simulink subsystem "Vehicle_plant_model"  (R2024b)
settings: Solver=VariableStepAuto  StartTime=0.0  StopTime=10.0  RelTol=1e-3
values from neighbouring files (symbols this model uses):
  div_min_MPC = 0.001    [sim_data_vehicle.sldd]    (also in sim_data_vehicle_nl.sldd)
  TimeStep = 0.01    [sim_data_DCmotor_system.sldd]    (also in sim_data_unstable_system.sldd = 0.01
undefined symbols (not defined in the file or in its folder): DiscIntNeverNeededParam, I_val, K_f_val, K_r_val, l_f_val, l_r_val, m_val, x0
settings Model: Creator=tshintai  LastModifiedBy=tshintai
settings SolverCC: AlgebraicLoopSolver=TrustRegion
settings OptimizationCC: ReuseModelBlockBuffer=off
settings DebuggingCC: UnconnectedInputMsg=warning  UnconnectedOutputMsg=warning  UnconnectedLineMsg=warning
settings ModelReferenceCC: EnableRefExpFcnMdlSchedulingChecks=on
settings RTWCC: GPUComputeCapability=3.5  DLArmComputeVersion=19.05

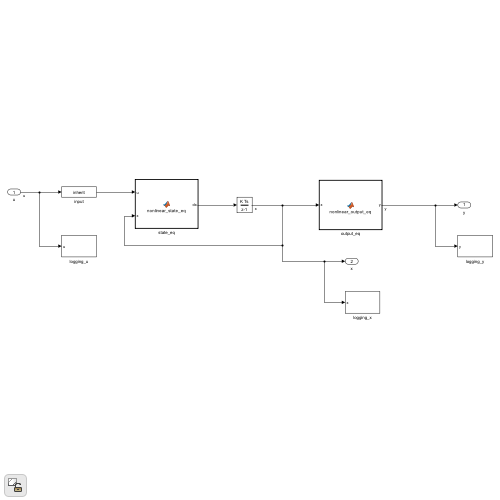
[thumbnail: Simulink's stored preview of the top-level diagram]
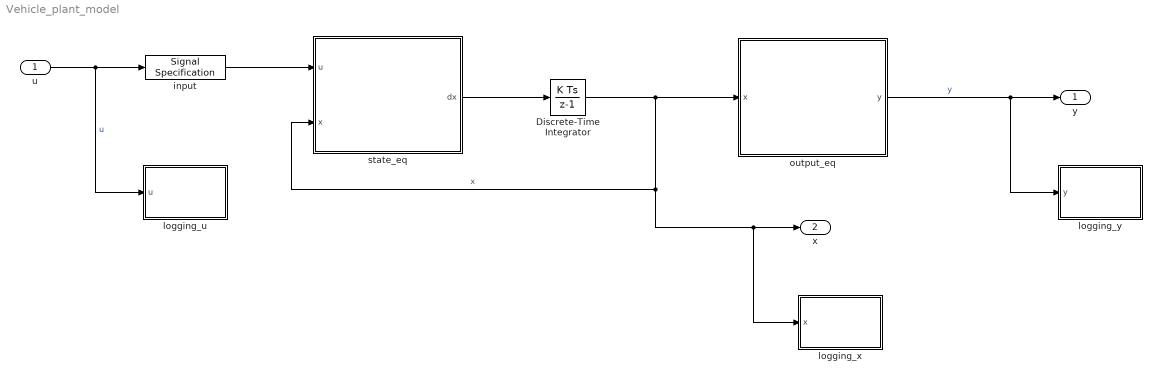
== system Vehicle_plant_model ==
  u : Inport
  Discrete-Time Integrator : DiscreteIntegrator  InitialCondition=x0  SampleTime=TimeStep  ICPrevOutput=DiscIntNeverNeededParam  ICPrevScaledInput=DiscIntNeverNeededParam
  input : SignalSpecification
  logging_u : Subsystem
  logging_x : Subsystem
  logging_y : Subsystem
  output_eq : MATLAB Function  TreatAsAtomicUnit=on
  state_eq : MATLAB Function  TreatAsAtomicUnit=on
  y : Outport
  x : Outport  Port=2
  wires:
  state_eq/1(dx) -> Discrete-Time Integrator/1
  u/1 -> input/1, logging_u/1(u)  "u"
  input/1 -> state_eq/1(u)
  output_eq/1(y) -> logging_y/1(y), y/1  "y"
  Discrete-Time Integrator/1 -> x/1, logging_x/1(x), state_eq/2(x), output_eq/1(x)  "x"

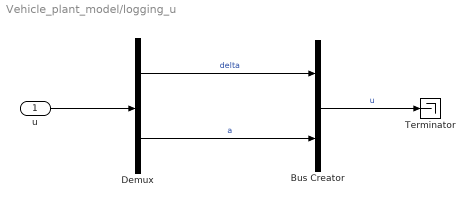
== system Vehicle_plant_model/logging_u ==
  u : Inport
  Bus Creator : BusCreator  Inputs=2
  Demux : Demux  Outputs=2
  Terminator : Terminator
  wires:
  Demux/1 -> Bus Creator/1  "delta"
  u/1 -> Demux/1
  Demux/2 -> Bus Creator/2  "a"
  Bus Creator/1 -> Terminator/1  "u"

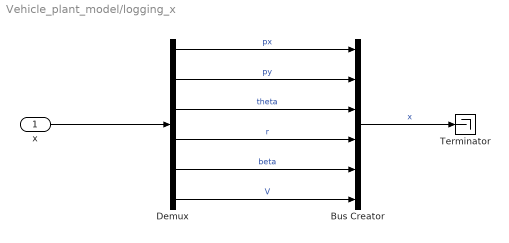
== system Vehicle_plant_model/logging_x ==
  x : Inport
  Bus Creator : BusCreator  Inputs=6
  Demux : Demux  Outputs=6
  Terminator : Terminator
  wires:
  Demux/6 -> Bus Creator/6  "V"
  Demux/3 -> Bus Creator/3  "theta"
  Demux/5 -> Bus Creator/5  "beta"
  Bus Creator/1 -> Terminator/1  "x"
  Demux/2 -> Bus Creator/2  "py"
  Demux/4 -> Bus Creator/4  "r"
  x/1 -> Demux/1
  Demux/1 -> Bus Creator/1  "px"

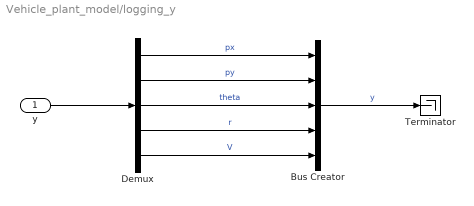
== system Vehicle_plant_model/logging_y ==
  y : Inport
  Bus Creator : BusCreator  Inputs=5
  Demux : Demux  Outputs=5
  Terminator : Terminator
  wires:
  Demux/1 -> Bus Creator/1  "px"
  y/1 -> Demux/1
  Demux/4 -> Bus Creator/4  "r"
  Demux/2 -> Bus Creator/2  "py"
  Bus Creator/1 -> Terminator/1  "y"
  Demux/5 -> Bus Creator/5  "V"
  Demux/3 -> Bus Creator/3  "theta"

== matlab function Vehicle_plant_model/state_eq ==
  data: u input; x input; dx output; I_val parameter; K_f_val parameter; K_r_val parameter; l_f_val parameter; l_r_val parameter; m_val parameter; div_min_MPC parameter
function dx = nonlinear_state_eq(u, x, I_val, K_f_val, K_r_val, ...
    l_f_val, l_r_val, m_val, div_min_MPC)

delta   = u(1);
a       = u(2);
theta   = x(3);
r       = x(4);
beta    = x(5);
V       = x(6);

% dx = calc_nonlinear_f(I_val, K_f_val, K_r_val, V, a, beta, delta, ...
%     l_f_val, l_r_val, m_val, r, theta);
dx = calc_nonlinear_f_azd(I_val, K_f_val, K_r_val, V, a, beta, delta, ...
    l_f_val, l_r_val, m_val, r, theta, div_min_MPC);

end

== matlab function Vehicle_plant_model/output_eq ==
  data: x input; y output; div_min_MPC parameter
function y = nonlinear_output_eq(x, div_min_MPC)

px      = x(1);
py      = x(2);
theta   = x(3);
r       = x(4);
V       = x(6);

% y = calc_nonlinear_h(V, px, py, r, theta);
y = calc_nonlinear_h_azd(V, px, py, r, theta, div_min_MPC);

end
